simulink model "Verifica_LQR_20042026"  (R2025b)
settings: Solver=VariableStepAuto  StartTime=0.0  StopTime=50.0  RelTol=1e-3
values from neighbouring files (symbols this model uses):
  A = double(subs(A_sym, [x; u], [x_star; u_star]))    [Main_20042026.m]
  B = double(subs(B_sym, [x; u], [x_star; u_star]))    [Main_20042026.m]
  C = double(subs(C_sym, [x; u], [x_star; u_star]))    [Main_20042026.m]
  D = double(subs(D_sym, [x; u], [x_star; u_star]))    [Main_20042026.m]
  h2_ref_lqr = 2.8    [Main_20042026.m]
  K_LQR_i = K_LQR(:, n+1:end)    [Main_20042026.m]
  K_LQR_x = K_LQR(:, 1:n)    [Main_20042026.m]
settings Model: Creator=salvo  LastModifiedBy=salvo

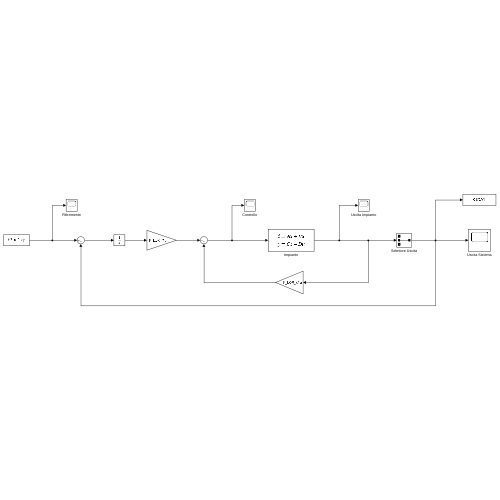
[thumbnail: Simulink's stored preview of the top-level diagram]
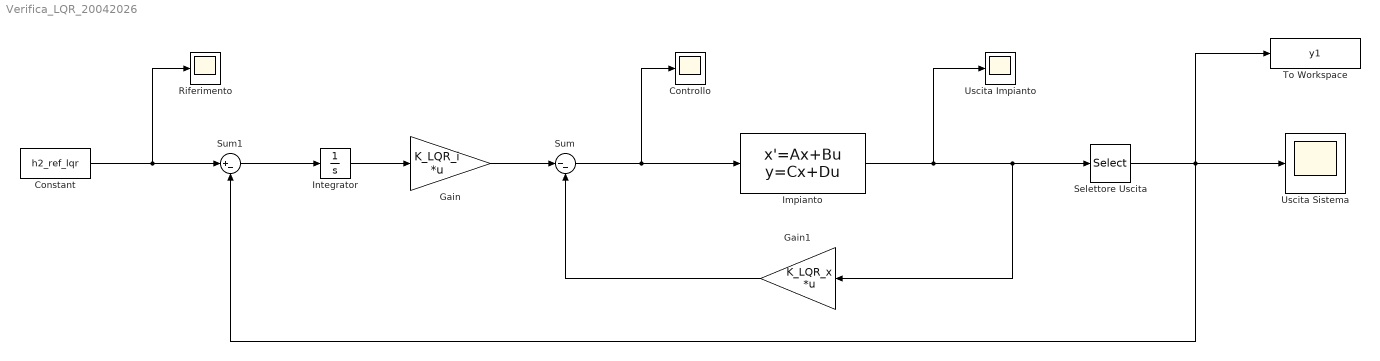
== system Verifica_LQR_20042026 ==
  Constant : Constant  Value=h2_ref_lqr
  Controllo : Scope
      settings: DataLoggingVariableName=ScopeData2
  Gain : Gain  Gain=K_LQR_i  Multiplication=Matrix(K*u)
  Gain1 : Gain  Gain=K_LQR_x  Multiplication=Matrix(K*u)
  Impianto : StateSpace  A=A  B=B  C=C  D=D  InitialCondition=0
  Integrator : Integrator
  Riferimento : Scope
  Selettore Uscita : Selector  InputPortWidth=3  IndexOptions=Index vector (dialog)  Indices=2  OutputSizes=1
  Sum : Sum  Inputs=|--
  Sum1 : Sum  Inputs=|+-
  To Workspace : ToWorkspace  VariableName=y1  SaveFormat=Timeseries  SampleTime=-1
  Uscita Impianto : Scope
      settings: DataLoggingVariableName=ScopeData3
  Uscita Sistema : Scope
      settings: ActiveDisplayYMinimum=1.8266267665549256  ActiveDisplayYMaximum=3.3536223642774354
  wires:
  Sum/1 -> Controllo/1, Impianto/1
  Impianto/1 -> Uscita Impianto/1, Selettore Uscita/1, Gain1/1
  Gain1/1 -> Sum/2
  Gain/1 -> Sum/1
  Integrator/1 -> Gain/1
  Sum1/1 -> Integrator/1
  Constant/1 -> Riferimento/1, Sum1/1
  Selettore Uscita/1 -> Sum1/2, To Workspace/1, Uscita Sistema/1
